simulink model "poly"  (R2015a)
settings: Solver=ode1  StartTime=0.0  StopTime=200  FixedStep=0.002  RelTol=1e-3
undefined symbols (not defined in the file): sigbuilder_block
settings Model: ExtModeTrigDuration=10000  Creator=bemran  LastModifiedBy=bemran
settings SolverCC: PositivePriorityOrder=on
settings RTWCC: SystemTargetFile=quarc_win64.tlc  TemplateMakefile=quarc_default_tmf  Description=QUARC Win64 Target
settings STFCustomTargetCC: TargetLibSuffix=.lib  TargetPreCompLibLocation=C:\PROGRA~3\QUARC\lib\2015a\win64\release  GenerateSampleERTMain=off  ConcurrentExecutionCompliant=on  GeneratePreprocessorConditionals=Disable all  ERTCustomFileBanners=off  SupportNonInlinedSFcns=on  SupportVariableSizeSignals=off  MATLABClassNameForMDSCustomization=Simulink.SoftwareTarget.GRTCustomization  GRTInterface=on  SystemTargetFile=quarc_win64.tlc
settings GRTTargetCC: TargetPreCompLibLocation=C:\PROGRA~3\QUARC\lib\2015a\win64\release  ParMdlRefBuildCompliant=off  CompOptLevelCompliant=off  CombineOutputUpdateFcns=off  MatFileLogging=off  CPPClassGenCompliant=off  GRTInterface=on  ExtMode=on  ExtModeMexFile=quarc_comm

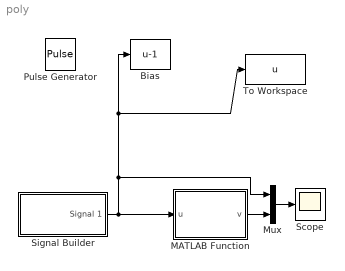
== system poly ==
  Bias : Bias  Bias=-1
  MATLAB Function : MATLAB Function  TreatAsAtomicUnit=on
  Mux : Mux  Inputs=2
  Pulse Generator : DiscretePulseGenerator  PulseType=Time based  Amplitude=0.6  PulseWidth=50
  Scope : Scope
      settings: TimeRange=200
  Signal Builder : Subsystem  Tag=STV Subsys  LoadFcn=sigbuilder_block('load');  StartFcn=sigbuilder_block('start');  StopFcn=sigbuilder_block('stop');  ClipboardFcn=sigbuilder_block('clipboard');  mask(Sigbuilder block){}
      mask help: Simulink:masks:SigbuilderBlock_MD
      mask init:
      | if ~strcmp(get_param(bdroot(gcbh),'SimulationStatus'),'stopped') tuvar = sigbuilder_block('maskInit'); end
      settings: CopyFcn=sigbuilder_block('copy');  DeleteFcn=sigbuilder_block('delete');  ModelCloseFcn=sigbuilder_block('modelClose');  PreSaveFcn=sigbuilder_block('preSave');  PauseFcn=sigbuilder_block('pause');  ContinueFcn=sigbuilder_block('continue');  NameChangeFcn=sigbuilder_block('namechange');  OpenFcn=sigbuilder_block('open',[437.6 199.2 550.4 400 ]);  CloseFcn=sigbuilder_block('close');
      mask Display: plot(0, 0, 100, 100,[2, 2, 32, 32, 2], [68, 8, 8, 68, 68],[32, 2], [38, 38], [32, 19, 2],[53, 60, 44], [32, 17, 17, 2],[16, 16, 31, 31]);txt = getActiveGroup(gcbh);text(2, 100, txt,'verticalAlignment', 'top');
  To Workspace : ToWorkspace  VariableName=u  SampleTime=-1
  wires:
  Signal Builder/1(Signal 1) -> To Workspace/1, Bias/1, Mux/1, MATLAB Function/1(u)
  MATLAB Function/1(v) -> Mux/2
  Mux/1 -> Scope/1

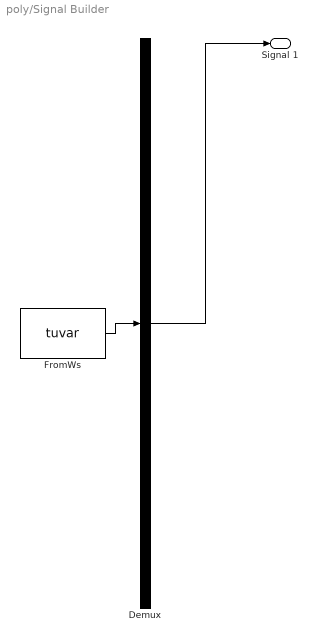
== system poly/Signal Builder ==
  Demux : Demux  Tag=STV Demux  Outputs=1
  FromWs : FromWorkspace  Tag=STV FromWs  VariableName=tuvar  SampleTime=0
      SigBuilderData=|
      | common.afterFinalStr = 'Extrapolate'
      | common.sampleTime = 0
      | dataSet.timeRange = [0 500]
      | dataSet.name = 'Group 1'
      | sbobj.Groups.Name = 'Group 1'
      | sbobj.Groups.Signals.Name = 'Signal 1'
      | sbobj.Groups.Signals.XData = [0 5 5 10 10 15 15 20 20 25 25 30 30 35 35 40 40 45 45 50 50 55 55 60 65 65 70 70 75 75 80 80 85 85 90 95 95 100 100 105 105 110 110 115 115 120 120 125 125 130 130 135 135 140 140 145 145 150 150 155 155 160 160 165 165 170 170 175 175 180 180 185 185 190 190 195 195 200 200 205 205 210 210 215 215 220 220 225 225 230 230 235 235 240 240 245 245 250 250 255 255 260 260 265 265 270 270 275 275 280 280 285 285 290 290 295 295 300 300 305 305 310 310 315 315 320 320 325 325 330 330 335 335 340 340 345 345 350 350 355 355 360 360 365 365 370 370 375 375 380 380 385 385 390 390 395 395 400 400 405 405 410 410 415 415 420 420 425 425 430 430 435 435 440 440 445 445 450 450 455 455 460 460 465 465 470 470 475 475 480 480 485 485 490 490 495 495 500]
      | sbobj.Groups.Signals.YData = [0.3 0.3 0 0 0.3 0.3 -0.3 -0.3 0 0 -0.3 -0.3 0.3 0.3 -0.3 -0.3 0 0 -0.3 -0.3 0.3 0.3 0 0 0 -0.3 -0.3 0 0 -0.3 -0.3 0.3 0.3 0 0 0 -0.3 -0.3 0.3 0.3 0 0 0.3 0.3 -0.3 -0.3 0.3 0.3 0 0 0.3 0.3 -0.3 -0.3 0.3 0.3 -0.3 -0.3 0 0 -0.3 -0.3 0 0 -0.3 -0.3 0.3 0.3 0 0 0.3 0.3 0 0 0.3 0.3 -0.3 -0.3 0.3 0.3 -0.3 -0.3 0.3 0.3 -0.3 -0.3 0.3 0.3 -0.3 -0.3 0.3 0.3 -0.3 -0.3 0.3 0.3 -0.3 -0.3 0.3 0.3 -0.3 -0.3 0.3 0.3 -0.3 -0.3 0.3 0.3 -0.3 -0.3 0.3 0.3 -0.3 -0.3 0.3 0.3 -0.3 -0.3 0.3 0.3 -0.3 -0.3 0.3 0.3 -0.3 -0.3 0.3 0.3 -0.3 -0.3 0.3 0.3 -0.3 -0.3 0.3 0.3 -0.3 -0.3 0.3 0.3 -0.3 -0.3 0.3 0.3 -0.3 -0.3 0.3 0.3 -0.3 -0.3 0.3 0.3 -0.3 -0.3 0.3 0.3 -0.3 -0.3 0.3 0.3 -0.3 -0.3 0.3 0.3 -0.3 -0.3 0.3 0.3 -0.3 -0.3 0.3 0.3 -0.3 -0.3 0.3 0.3 -0.3 -0.3 0.3 0.3 -0.3 -0.3 0.3 0.3 -0.3 -0.3 0.3 0.3 -0.3 -0.3 0.3 0.3 -0.3 -0.3 0.3 0.3 -0.3 -0.3]
      | sbobj.Groups.TimeRange = [0 500]
  Signal 1 : Outport  Tag=STV Outport
  wires:
  Demux/1 -> Signal 1/1
  FromWs/1 -> Demux/1

== matlab function poly/MATLAB Function ==
  data: u input; v output
function v = fcn(u)
%#codegen
persistent v0 u0

if isempty(u0)
    u0 = 0;
    v0 = 0;
end
if (u == 0)
    v = 0;
else
    v = v0 + u - 0.9998 * u0;
end
v0 = v;
u0 = u;
